simulink model "sem1_assignment"  (R2021b)
settings: Solver=VariableStepAuto  StartTime=0.0  StopTime=10  RelTol=1e-3
libraries: simulink_extras x4, SignalEditorBlockLib x3, hdlsllib x1
settings Model: Creator=l_tan  LastModifiedBy=l_tan

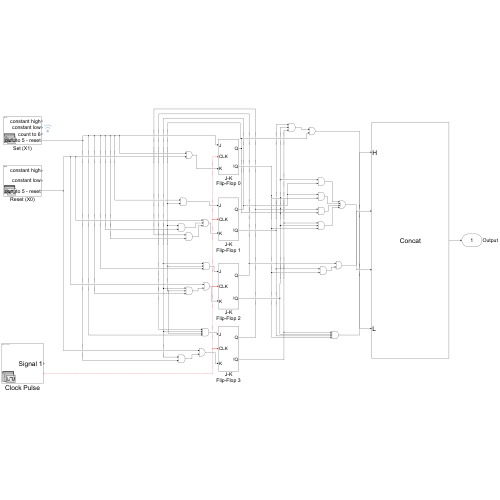
[thumbnail: Simulink's stored preview of the top-level diagram]
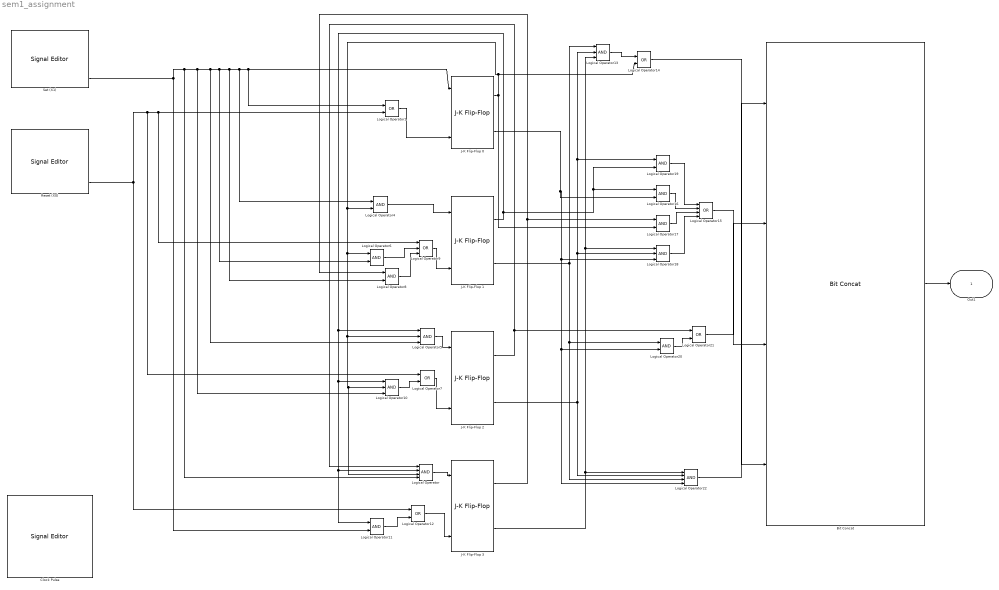
== system sem1_assignment ==
  Bit Concat : hdlsllib/Logic and Bit Operations/Bit Concat  numInputs=4
  Clock Pulse : SignalEditorBlockLib/Signal Editor  FileName=C:\Users\l_tan\Documents\Year 2 uni\EE270\semester 1 assignment\high.mat  ActiveScenario=Scenario  ActiveSignal=high  IsBus=off  OutputBusObjectStr=Bus: BusObject  SampleTime=0  Interpolate=off  ZeroCross=off  OutputAfterFinalValue=Setting to zero  Unit=inherit  PreserveSignalName=on
  J-K Flip-Flop {0..3} (4 alike) : simulink_extras/Flip Flops/J-K Flip-Flop  initial_condition=0
  Logical Operator : Logic  Inputs=4  IconShape=distinctive  AllPortsSameDT=off  OutDataTypeStr=boolean
  Logical Operator{1,7,12,14,21} (5 alike) : Logic  Operator=OR  IconShape=distinctive  AllPortsSameDT=off  OutDataTypeStr=boolean
  Logical Operator{5,10,13,18} (4 alike) : Logic  Inputs=3  IconShape=distinctive  AllPortsSameDT=off  OutDataTypeStr=boolean
  Logical Operator{4,6,8,11,16..17,19..20} (8 alike) : Logic  IconShape=distinctive  AllPortsSameDT=off  OutDataTypeStr=boolean
  Logical Operator15 : Logic  Operator=OR  Inputs=4  IconShape=distinctive  AllPortsSameDT=off  OutDataTypeStr=boolean
  Logical Operator22 : Logic  Inputs=4  IconShape=distinctive  AllPortsSameDT=off  OutDataTypeStr=boolean
  Logical Operator9 : Logic  Operator=OR  Inputs=3  IconShape=distinctive  AllPortsSameDT=off  OutDataTypeStr=boolean
  Reset (X0) : SignalEditorBlockLib/Signal Editor  FileName=C:\Users\l_tan\Documents\Year 2 uni\EE270\semester 1 assignment\X0_tests.mat  ActiveScenario=X0  ActiveSignal=constant high  IsBus=off  OutputBusObjectStr=Bus: BusObject  SampleTime=0  Interpolate=off  ZeroCross=off  OutputAfterFinalValue=Setting to zero  Unit=inherit  PreserveSignalName=on
  Set (X1) : SignalEditorBlockLib/Signal Editor  FileName=C:\Users\l_tan\Documents\Year 2 uni\EE270\semester 1 assignment\X1_tests.mat  ActiveScenario=X1  ActiveSignal=constant high  IsBus=off  OutputBusObjectStr=Bus: BusObject  SampleTime=0  Interpolate=off  ZeroCross=off  OutputAfterFinalValue=Setting to zero  Unit=inherit  PreserveSignalName=on
  Out1 : Outport  SignalName=Output
  wires:
  Logical Operator/1 -> J-K Flip-Flop 3/1
  Logical Operator5/1 -> J-K Flip-Flop 2/1
  Logical Operator7/1 -> J-K Flip-Flop 2/3
  Set (X1)/4 -> Logical Operator/4, Logical Operator10/3, Logical Operator5/3, Logical Operator6/2, Logical Operator1/1, J-K Flip-Flop 0/1, Logical Operator4/1, Logical Operator8/2, Logical Operator11/2
  Logical Operator1/1 -> J-K Flip-Flop 0/3
  Logical Operator4/1 -> J-K Flip-Flop 1/1
  J-K Flip-Flop 0/1 -> Logical Operator17/2, Logical Operator/3, Logical Operator10/2, Logical Operator5/2, Logical Operator6/1, Logical Operator4/2, Logical Operator14/2
  Logical Operator9/1 -> J-K Flip-Flop 1/3
  J-K Flip-Flop 3/1 -> Logical Operator17/1, Logical Operator8/1
  Logical Operator6/1 -> Logical Operator9/2
  Logical Operator8/1 -> Logical Operator9/3
  J-K Flip-Flop 1/1 -> Logical Operator11/1, Logical Operator/2, Logical Operator10/1, Logical Operator5/1, Logical Operator16/1, Logical Operator19/2
  Logical Operator10/1 -> Logical Operator7/2
  Reset (X0)/3 -> Logical Operator7/1, Logical Operator9/1, Logical Operator1/2, Logical Operator12/1
  J-K Flip-Flop 2/1 -> Logical Operator/1, Logical Operator21/1
  Logical Operator11/1 -> Logical Operator12/2
  Logical Operator12/1 -> J-K Flip-Flop 3/3
  J-K Flip-Flop 3/2 -> Logical Operator22/1, Logical Operator18/1, Logical Operator13/3
  J-K Flip-Flop 2/2 -> Logical Operator18/2, Logical Operator19/1, Logical Operator13/2, Logical Operator22/2
  J-K Flip-Flop 1/2 -> Logical Operator13/1, Logical Operator20/1, Logical Operator22/3
  Logical Operator13/1 -> Logical Operator14/1
  Logical Operator14/1 -> Bit Concat/4
  J-K Flip-Flop 0/2 -> Logical Operator16/2, Logical Operator18/3, Logical Operator22/4, Logical Operator20/2
  ? -> J-K Flip-Flop 3/2, J-K Flip-Flop 2/2, J-K Flip-Flop 0/2, J-K Flip-Flop 1/2
  Logical Operator15/1 -> Bit Concat/3
  Logical Operator18/1 -> Logical Operator15/4
  Logical Operator17/1 -> Logical Operator15/3
  Logical Operator16/1 -> Logical Operator15/2
  Logical Operator19/1 -> Logical Operator15/1
  Logical Operator20/1 -> Logical Operator21/2
  Logical Operator22/1 -> Bit Concat/1
  Bit Concat/1 -> Out1/1
  Logical Operator21/1 -> Bit Concat/2
